simulink model "boost_switching"  (Simulink 6.5)
settings: Solver=ode45  StartTime=0.0  StopTime=10000e-6  MaxStep=0.1e-6  RelTol=1e-3
libraries: simulink x1
settings Model: Creator=Mama  LastModifiedBy=Dragan Maksimovic
settings DebuggingCC: AlgebraicLoopMsg=none  SolverPrmCheckMsg=none  UnconnectedOutputMsg=none

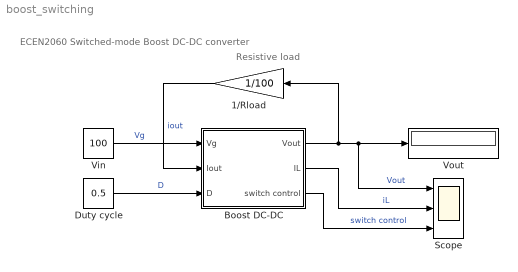
== system boost_switching ==
  note: ECEN2060
      | Switched-mode Boost
      | DC-DC converter
  note: Resistive load
  1/Rload : Gain  Orientation=left  Gain=1/100
  Boost DC-DC : Subsystem  mask{L=200e-6, Io=4, C=10e-6, Vo=200, fs=100e3}
      mask prompts: L "Inductance"; Io "Initial inductor current"; C "Capacitance"; Vo "Initial capacitor voltage"; fs "Switching frequency"
      mask help: Switched-mode Boost (step-up) DC-DC converter (switching). The duty-cycle D determines the step-up voltage conversion ratio, Vout/Vg = 1/(1-D). The model is ideal, losses are neglected, efficiency is 100%
      mask Display:
      | text(0.5,0.75,'Boost','horizontalAlignment', 'center');
      | text(0.5,0.6,'DC-DC','horizontalAlignment', 'center');
      | text(0.5,0.45,'(switching)','horizontalAlignment', 'center');
  Duty cycle : Constant  Value=0.5  OutDataType=sfix(16)  ConRadixGroup=Use specified scaling  OutScaling=2^0  SampleTime=inf  FramePeriod=inf
  Scope : Scope  NumInputPorts=3
      settings: TimeRange=0.01  YMin=180~0~-0.5  YMax=220~8~1.5
  Vin : Constant  Value=100  OutDataType=sfix(16)  ConRadixGroup=Use specified scaling  OutScaling=2^0  SampleTime=inf  FramePeriod=inf
  Vout : Display
  wires:
  Duty cycle/1 -> Boost DC-DC/3(D)  "D"
  Vin/1 -> Boost DC-DC/1(Vg)  "Vg"
  Boost DC-DC/1(Vout) -> Vout/1, Scope/1, 1/Rload/1  "Vout"
  Boost DC-DC/2(IL) -> Scope/2  "iL"
  Boost DC-DC/3(switch control) -> Scope/3  "switch control"
  1/Rload/1 -> Boost DC-DC/2(Iout)  "iout"

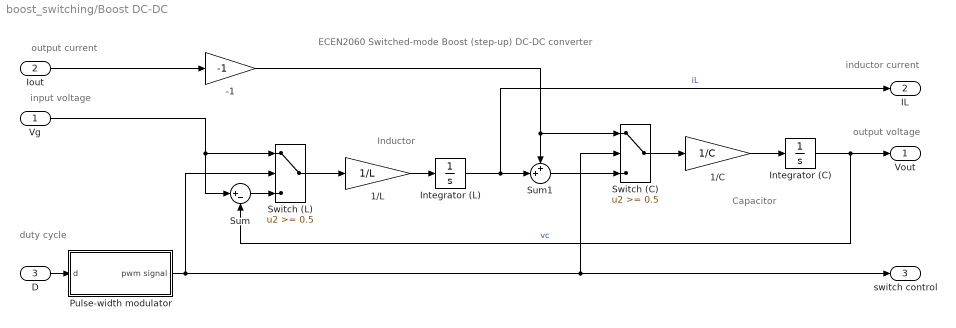
== system boost_switching/Boost DC-DC ==
  note: ECEN2060 Switched-mode Boost (step-up) DC-DC converter
  note: output voltage
  note: inductor current
  note: output current
  note: input voltage
  note: duty cycle
  note: Inductor
  note: Capacitor
  Vg : Inport
  Iout : Inport  Port=2
  D : Inport  Port=3
  -1 : Gain  Gain=-1
  1/C : Gain  Gain=1/C
  1/L : Gain  Gain=1/L
  Integrator (C) : Integrator  InitialCondition=Vo
  Integrator (L) : Integrator  InitialCondition=Io
  Pulse-width modulator : Subsystem  mask{Fs=fs}
      mask prompts: Fs "Switching frequency"
  Sum : Sum  Inputs=|+-
  Sum1 : Sum  Inputs=++|
  Switch (C) : Switch  Threshold=0.5
  Switch (L) : Switch  Threshold=0.5
  Vout : Outport
  IL : Outport  Port=2
  switch control : Outport  Port=3
  wires:
  Vg/1 -> Switch (L)/1, Sum/1
  Pulse-width modulator/1(pwm signal) -> Switch (L)/2, Switch (C)/2, switch control/1
  Sum/1 -> Switch (L)/3
  Sum1/1 -> Switch (C)/3
  Switch (C)/1 -> 1/C/1
  1/C/1 -> Integrator (C)/1
  Integrator (C)/1 -> Sum/2, Vout/1  "vc"
  Switch (L)/1 -> 1/L/1
  1/L/1 -> Integrator (L)/1
  Integrator (L)/1 -> Sum1/2, IL/1  "iL"
  D/1 -> Pulse-width modulator/1(d)
  Iout/1 -> -1/1
  -1/1 -> Sum1/1, Switch (C)/1

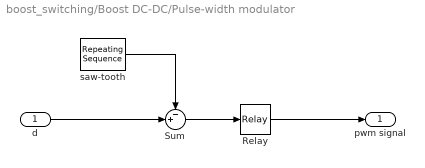
== system boost_switching/Boost DC-DC/Pulse-width modulator ==
  d : Inport
  Relay : Relay
  Sum : Sum  Inputs=-+|
  saw-tooth : simulink/Sources/Repeating Sequence  SystemSampleTime=-1  rep_seq_t=[0 1/Fs]  rep_seq_y=[0 1]
  pwm signal : Outport
  wires:
  d/1 -> Sum/2
  saw-tooth/1 -> Sum/1
  Sum/1 -> Relay/1
  Relay/1 -> pwm signal/1
